simulink model "sl_subsys_fcncallerr6"  (Simulink 6.0)
settings: Solver=FixedStepDiscrete  StartTime=0.0  StopTime=10.0  FixedStep=1  RelTol=1e-3
settings Model: CovMetricSettings=d  Creator=The MathWorks Inc.  LastModifiedBy=batserve  ExtModeAutoUpdateStatusClock=off
settings OptimizationCC: BlockReduction=off  BooleanDataType=off
settings DebuggingCC: CheckExecutionContextPreStartOutputMsg=on  CheckExecutionContextRuntimeOutputMsg=on  SolverPrmCheckMsg=none
settings HardwareCC: TargetUnknown=on

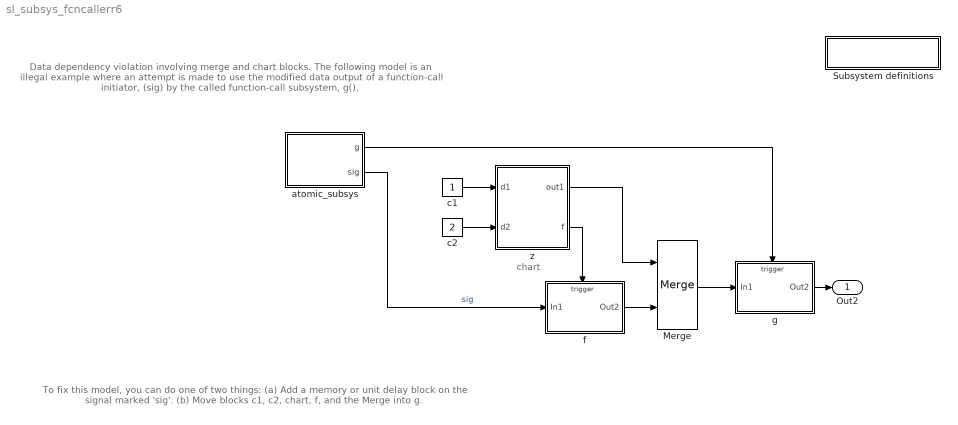
== system sl_subsys_fcncallerr6 ==
  note: To fix this model, you can do one of two things:
      | (a) Add a memory or unit delay block on the signal marked 'sig'.
      | (b) Move blocks c1, c2, chart, f, and the Merge into g.
  note: Data dependency violation involving merge and chart blocks.
      |
      | The following model is an illegal example where an attempt is made
      | to use the modified data output of a function-call initiator, (sig)
      | by the called function-call subsystem, g().
  note: chart
  " Subsystem definitions" : Subsystem  PropExecContextAcrossSSBoundary=on
      settings: OpenFcn=helpview([matlabroot,'/toolbox/simulink/simdemos/sl_subsys_definitions.html']);
      mask Display: disp('Subsystem\ndefinitions')
  Merge : Merge
  atomic_subsys : Subsystem  TreatAsAtomicUnit=on  PropExecContextAcrossSSBoundary=on
  c1 : Constant
  c2 : Constant  Value=2
  f : Subsystem  TreatAsAtomicUnit=on  PropExecContextAcrossSSBoundary=on
  g : Subsystem  TreatAsAtomicUnit=on  PropExecContextAcrossSSBoundary=on
  z : Stateflow chart  PropExecContextAcrossSSBoundary=on
  Out2 : Outport
  wires:
  z/2(f) -> f/Trigger
  atomic_subsys/1(g) -> g/Trigger
  f/1(Out2) -> Merge/2
  Merge/1 -> g/1(In1)
  z/1(out1) -> Merge/1
  atomic_subsys/2(sig) -> f/1(In1)  "sig"
  c1/1 -> z/1(d1)
  c2/1 -> z/2(d2)
  g/1(Out2) -> Out2/1

== system sl_subsys_fcncallerr6/ Subsystem definitions ==

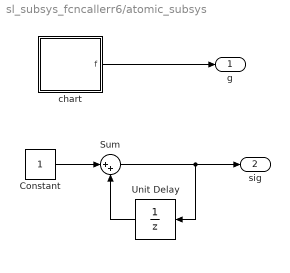
== system sl_subsys_fcncallerr6/atomic_subsys ==
  Constant : Constant
  Sum : Sum  Inputs=|++  SaturateOnIntegerOverflow=on  InputSameDT=on
  Unit Delay : UnitDelay  Orientation=left  SampleTime=-1
  chart : Stateflow chart  PropExecContextAcrossSSBoundary=on
  g : Outport
  sig : Outport  Port=2
  wires:
  chart/1(f) -> g/1
  Sum/1 -> sig/1, Unit Delay/1
  Constant/1 -> Sum/1
  Unit Delay/1 -> Sum/2

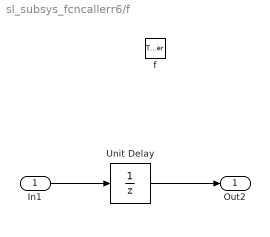
== system sl_subsys_fcncallerr6/f ==
  In1 : Inport  Port=1  LatchInput=off
  f : TriggerPort  TriggerType=function-call
  Unit Delay : UnitDelay  SampleTime=-1
  Out2 : Outport
  wires:
  In1/1 -> Unit Delay/1
  Unit Delay/1 -> Out2/1

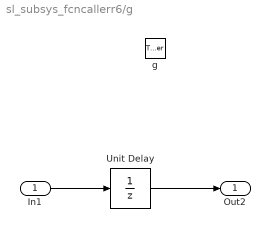
== system sl_subsys_fcncallerr6/g ==
  In1 : Inport  Port=1  LatchInput=off
  g : TriggerPort  TriggerType=function-call
  Unit Delay : UnitDelay  SampleTime=-1
  Out2 : Outport
  wires:
  In1/1 -> Unit Delay/1
  Unit Delay/1 -> Out2/1

== stateflow chart z ==
  state one/
    entry:f;out1=d1+d2;
  state two/
    entry: f;out1=d1-d2;
  one -> two
  two -> one
  (default) -> one
  data: d1 input double; d2 input double; out1 output double; out local double
  events: f output FUNCTION_CALL_EVENT

== stateflow chart atomic_subsys/chart ==
  state one/
    entry: f;
  state two/
    entry: f;
  one -> two
  two -> one
  (default) -> one
  events: f output FUNCTION_CALL_EVENT
